simulink model "simu"  (R2019b)
settings: Solver=VariableStepAuto  StartTime=0.0  StopTime=inf  RelTol=1e-3
InitFcn:
  | Workspace
StopFcn:
  | save('myvars.mat','out')
  | plotmyvars
model workspace: external: MATLAB File E:\0-数理基础\A-数\00MATLAB\B-仿真分析\0-理解Simulink机制\MSA\simulinkpara.m (data not in the file)
values from neighbouring files (symbols this model uses):
  c = 10    [Workspace.m]
settings Model: Creator=wdther  LastModifiedBy=wdther

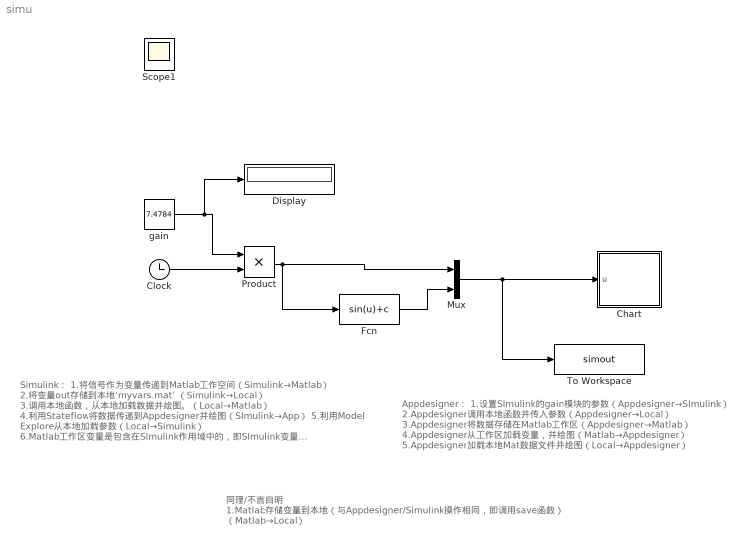
== system simu ==
  note: 同理/不言自明
      | 1.Matlab存储变量到本地（与Appdesigner/Simulink操作相同，即调用save函数）
      | （Matlab→Local）
  note: Appdesigner：
      | 1.设置SImulink的gain模块的参数（Appdesigner→SImulink）
      | 2.Appdesigner调用本地函数并传入参数（Appdesigner→Local）
      | 3.Appdesigner将数据存储在Matlab工作区（Appdesigner→Matlab）
      | 4.Appdesigner从工作区加载变量，并绘图（Matlab→Appdesigner）
      | 5.Appdesigner加载本地Mat数据文件并绘图（Local→Appdesigner）
  note: Simulink：
      | 1.将信号作为变量传递到Matlab工作空间（Simulink→Matlab）
      | 2.将变量out存储到本地‘myvars.mat’ （Simulink→Local）
      | 3.调用本地函数，从本地加载数据并绘图。（Local→Matlab）
      | 4.利用Stateflow将数据传递到Appdesigner并绘图（SImulink→App）
      | 5.利用Model Explore从本地加载参数（Local→Simulink）
      | 6.Matlab工作区变量是包含在SImulink作用域中的，即SImulink变量
      | 可以随意调用Matlab工作区变量,图中sin(u)+c所示（Matlab→Simulink）
  Chart : Stateflow chart  BlockKeywords=__PRM__SERIALIZED__DATA__:Stateflow Chart,Stateflow Diagram  TreatAsAtomicUnit=on
  Clock : Clock
  Display : Display
  Fcn : Fcn  Expr=sin(u)+c
  Mux : Mux  Inputs=2
  Product : Product
  To Workspace : ToWorkspace  VariableName=simout  SampleTime=-1
      settings: Save2DSignal=2-D array (concatenate along first dimension)
  gain : Constant  Value=7.4784
  Scope1 : Scope
  wires:
  Clock/1 -> Product/2
  Mux/1 -> Chart/1(u), To Workspace/1
  Fcn/1 -> Mux/2
  gain/1 -> Display/1, Product/1
  Product/1 -> Fcn/1, Mux/1

== stateflow chart simu/Chart ==
  state INIT
    en:
    coder.extrinsic('App','plotxy')
    app=App();
  state Plot
    du:
    X=u(1); %取第一列数据
    Y=u(2);
    plotxy(app,X,Y);
  (default) -> INIT
  INIT -> Plot
  data: u input; X local; Y local; app local
